simulink model "sequenceprueba"  (R2021b)
settings: Solver=VariableStepAuto  StartTime=0.0  StopTime=10.0  RelTol=1e-3
values from neighbouring files (symbols this model uses):
  fp = [t1;t2;t3]    [creacionestructurasborrador.m]    (also in flight_plan.m = [sid,wps,iap]; flight_plan_eval.m = [t1;tabla2;t3]; flight_plan_old.m = [sid,wps,iap]; flight_plan_struct.m = [t1;tabla2;t3])
  tabla4 = table2struct(tabla4)    [creacionestructurasborrador.m]
libraries: simulink x1
settings Model: Creator=verti  LastModifiedBy=verti

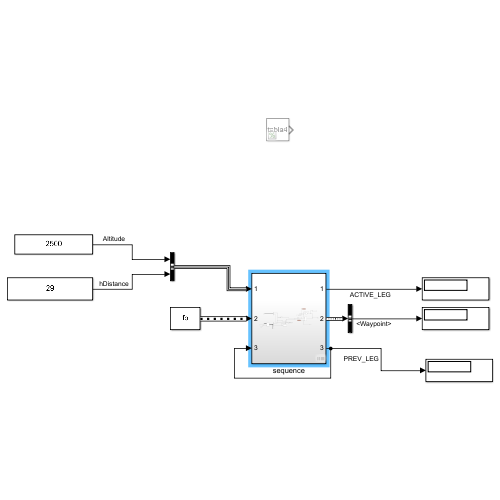
[thumbnail: Simulink's stored preview of the top-level diagram]
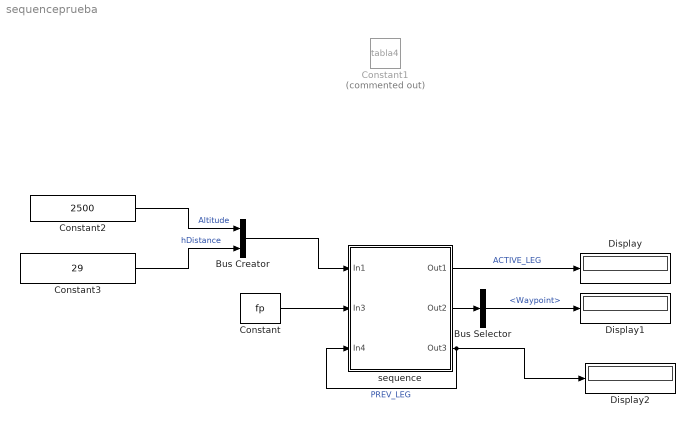
== system sequenceprueba ==
  Bus Creator : BusCreator  Inputs=2
  Bus Selector : BusSelector  OutputSignals=Waypoint
  Constant : Constant  Value=fp  OutDataTypeStr=Bus: BUS_FP
  Constant1 : Constant  Commented=on  Value=tabla4  OutDataTypeStr=Bus: BUS_ACTUAL
  Constant2 : Constant  Value=2500
  Constant3 : Constant  Value=29
  Display : Display
  Display1 : Display
  Display2 : Display
  sequence : Subsystem
  wires:
  sequence/3(Out3) -> sequence/3(In4), Display2/1  "PREV_LEG"
  Constant3/1 -> Bus Creator/2  "hDistance"
  Constant2/1 -> Bus Creator/1  "Altitude"
  Bus Creator/1 -> sequence/1(In1)
  Constant/1 -> sequence/2(In3)
  sequence/1(Out1) -> Display/1  "ACTIVE_LEG"
  sequence/2(Out2) -> Bus Selector/1
  Bus Selector/1 -> Display1/1  "<Waypoint>"

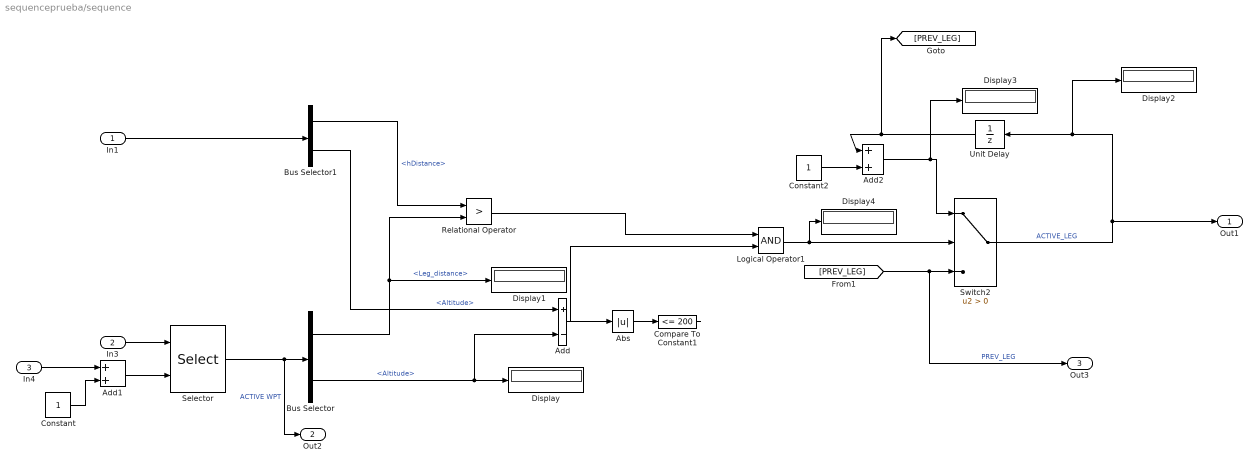
== system sequenceprueba/sequence ==
  In1 : Inport  RequirementInfo={} %GIDa_c5110965_b51e_4bd0_aaf9_593ecd07351e
  In3 : Inport  RequirementInfo={} %GIDa_249b9ffc_5b09_4262_affd_d906ea8e163e  Port=2
  In4 : Inport  RequirementInfo={} %GIDa_5bd288b4_a1e1_4c2e_8550_56976680c4ff  Port=3
  Abs : Abs  RequirementInfo={} %GIDa_c7b76162_8267_4ca6_b227_9716dada5505
  Add : Sum  RequirementInfo={} %GIDa_1f565a9c_bb6c_4277_a15a_2dd9ddc74e2c  Inputs=+-
  Add1 : Sum
  Add2 : Sum  RequirementInfo={} %GIDa_10ba33e9_01e3_419e_92f2_df268cced54e
  Bus Selector : BusSelector  RequirementInfo={} %GIDa_32044838_e93b_4295_a6ba_56cafa775409  OutputSignals=Leg_distance,Altitude
  Bus Selector1 : BusSelector  RequirementInfo={} %GIDa_ba4ca1dd_ac53_495e_9fd0_7384afdc2a56  OutputSignals=hDistance,Altitude
  Compare To Constant1 : simulink/Logic and Bit Operations/Compare To Constant  RequirementInfo={} %GIDa_08ea8b3d_3662_4990_84e4_c4fe850e2295  relop=<=  const=200  OutDataTypeStr=boolean
  Constant : Constant
  Constant2 : Constant  RequirementInfo={} %GIDa_2a6fc1af_ea43_468a_b994_1ceeebaeb3ce
  Display{,1..4} (5 alike) : Display
  Logical Operator1 : Logic  RequirementInfo={} %GIDa_87c16c20_fd62_4a0f_bcd6_f1e5af88d04d  AllPortsSameDT=off  OutDataTypeStr=boolean
  Relational Operator : RelationalOperator  RequirementInfo={} %GIDa_5ebf44e6_f006_46ab_96ba_7ababa2b4cc8  Operator=>  OutDataTypeStr=boolean  RndMeth=Simplest
  Selector : Selector  RequirementInfo={} %GIDa_dce26692_3f36_4dca_befe_722dd4cf467c  InputPortWidth=12  IndexOptions=Index vector (port)  Indices=[1 3]  OutputSizes=1
  Switch2 : Switch  RequirementInfo={} %GIDa_32b6e294_5707_4454_a8d7_32d9b5fe67d4  Criteria=u2 > Threshold
  Unit Delay : UnitDelay  RequirementInfo={} %GIDa_e6305557_f123_4806_b72d_76220e49e1a9  SampleTime=-1  HasFrameUpgradeWarning=on
  Out1 : Outport  RequirementInfo={} %GIDa_f72c117e_f023_4828_99ec_20f9b203fad8
  Out2 : Outport  RequirementInfo={} %GIDa_1093e2f4_6b11_4d8f_8352_e6ef1b08730a  Port=2
  Out3 : Outport  RequirementInfo={} %GIDa_d3bcf687_f8b9_4ce1_b3bb_1ad8d3769b6f  Port=3
  wires:
  Selector/1 -> Out2/1, Bus Selector/1  "ACTIVE WPT"
  In4/1 -> Add1/1
  Add/1 -> Abs/1
  In3/1 -> Selector/1
  Constant2/1 -> Add2/2
  Unit Delay/1 -> Add2/1, [PREV_LEG]
  Bus Selector1/1 -> Relational Operator/1  "<hDistance>"
  Bus Selector/1 -> Display1/1, Relational Operator/2  "<Leg_distance>"
  Logical Operator1/1 -> Display4/1, Switch2/2
  Bus Selector/2 -> Add/2, Display/1  "<Altitude>"
  Abs/1 -> Compare To Constant1/1
  In1/1 -> Bus Selector1/1
  Bus Selector1/2 -> Add/1  "<Altitude>"
  Compare To Constant1/1 -> Logical Operator1/2
  Add2/1 -> Display3/1, Switch2/1
  [PREV_LEG] -> Switch2/3, Out3/1  "PREV_LEG"
  Switch2/1 -> Out1/1, Display2/1, Unit Delay/1  "ACTIVE_LEG"
  Relational Operator/1 -> Logical Operator1/1
  Add1/1 -> Selector/2
  Constant/1 -> Add1/2
